simulink model "main"  (R2025b)
settings: Solver=FixedStepDiscrete  StartTime=0.0  StopTime=Inf  RelTol=1e-3  EnableMultiTasking=on
PreLoadFcn:
  | RTWConfigurationCB('preloadfcn', bdroot);
model workspace (MAT data in the model file):
  fault_count = 0
  fz_values = [0 50 100 150 200 250 300 350 400 450 500 550 600 650 700 750 800 850 900 950 1000 1050 1100 1150 1200 1250 1300 1350 1400 1450 1500 1550 1600 1650 1700 1750 1800 1850 1900 1950 2000 2050 2100]
  k_opt_lut = [0 0 0 0 0 0 0 0 0 0 0 0 ... (4386 elements, 51x2x43)]
  mu_opt_lut = [0 0 0 0 0 0 0 0 0 0 0 0 ... (4386 elements, 51x2x43)]
undefined symbols (not defined in the file or in its folder): bit, Call, Function, ocv_lut, slope_lut, soc_lut
libraries: c2837xDlib x34, c280xlib x20, canmsglib x18, c2802xlib x12, simulink x9, slpidlib x3
(part 1 of 5)
settings Model: SimulationMode=external  ExtModeTrigDuration=8  Creator=Brian  LastModifiedBy=levin
settings SolverCC: AutoInsertRateTranBlk=on
settings OptimizationCC: DefaultParameterBehavior=Inlined  DefaultUnderspecifiedDataType=single  EnhancedBackFolding=on  PassReuseOutputArgsAs=Individual arguments  MaxStackSize=1024  OptimizeBlockOrder=speed  DifferentSizesBufferReuse=on  OptimizationCustomize=off  DenormalBehavior=FlushToZero  EfficientTunableParamExpr=on
settings DebuggingCC: ParameterTunabilityLossMsg=error
settings HardwareCC: ProdBitPerChar=16.0  ProdBitPerInt=16.0  ProdBitPerPointer=32.0  ProdBitPerSizeT=32.0  ProdBitPerPtrDiffT=32.0  ProdLargestAtomicInteger=Integer  ProdLargestAtomicFloat=None  ProdWordSize=16.0  ProdLongLongMode=on  ProdHWDeviceType=Texas Instruments->C2000  HardwareBoardFeatureSet=SoCBlockset
settings ModelReferenceCC: EnableRefExpFcnMdlSchedulingChecks=on  ModelReferenceNumInstancesAllowed=Single
settings SFSimCC: MATLABDynamicMemAlloc=off
settings RTWCC: SystemTargetFile=ert.tlc  HardwareBoard=TI Delfino F28379D LaunchPad  TemplateMakefile=ert_default_tmf  Toolchain=Texas Instruments Code Composer Studio (C2000)  CodeProfilingSaveOptions=MetricsOnly  GPUComputeCapability=3.5  Description=Embedded Coder
settings CodeAppCC: ForceParamTrailComments=on  IgnoreCustomStorageClasses=off  OperatorAnnotations=on  SimulinkDataObjDesc=on  SFDataObjDesc=on  InsertBlockDesc=on
settings ERTTargetCC: ExtModeTransport=4.0  ExtModeStaticAlloc=on  ExtModeAutomaticAllocSize=off  ExtModeStaticAllocSize=10000.0  ExtModeMexFile=ext_xcp  ExtModeIntrfLevel=Level2 - Open  InlinedParameterPlacement=Hierarchical  DynamicArrayContainerType=coder::array  CodeReplacementLibrary=TI C28x  SubcomponentCodeInterfacePackaging=Nonreusable function

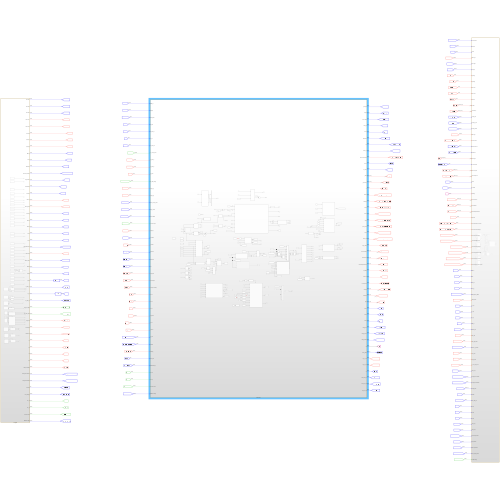
[thumbnail: Simulink's stored preview of the top-level diagram]
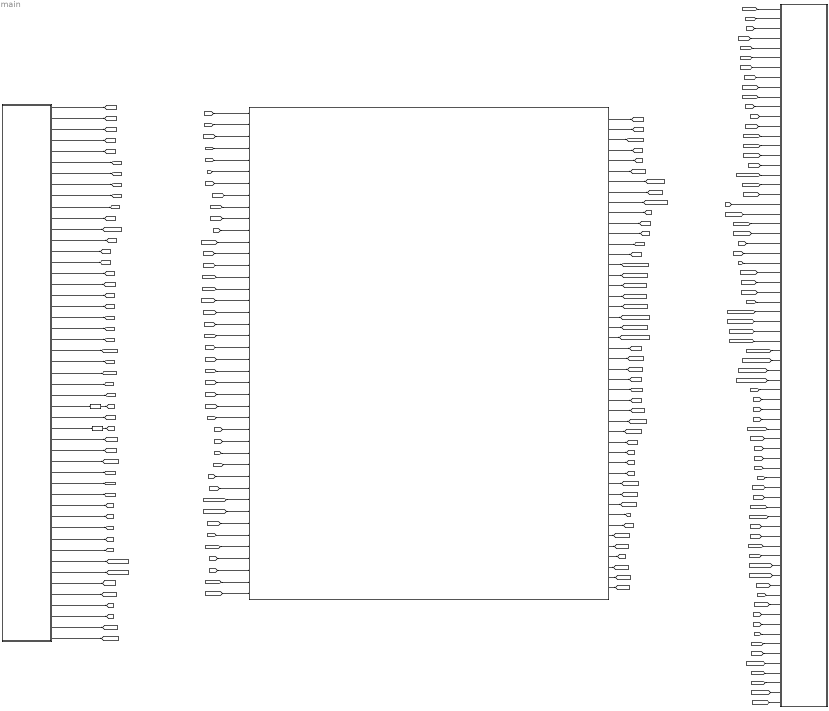
== system main ==
  Cast To Double2 : DataTypeConversion  OutDataTypeStr=uint16  SaturateOnIntegerOverflow=off  RndMeth=Floor
  Cast To Double4 : DataTypeConversion  OutDataTypeStr=uint16  SaturateOnIntegerOverflow=off  RndMeth=Floor
  In Signals : Subsystem
  MCU Code : Subsystem
  Subsystem : Subsystem
  wires:
  In Signals/5(BPT Front 2) -> [bpt_front_2]
  In Signals/20(BPT OC) -> [BPT_OC]
  In Signals/24(BSPD Fault) -> [BSPD_FAULT]
  In Signals/36(Lateral Accel) -> [Lat_Accel]
  In Signals/39(RL) -> [wss_rl]
  In Signals/29(ts_state_len) -> [ts_state_len]
  In Signals/25(Start Up Active) -> [START_UP_ACTIVE]
  In Signals/28(ts_state) -> Cast To Double2/1
  In Signals/38(FR) -> [wss_fr]
  In Signals/31(inv_state_len) -> [inv_state_len]
  In Signals/26(BMS IN) -> [BMS_IN]
  In Signals/33(inv_motor_speed) -> [inv_motor_speed]
  In Signals/40(RR) -> [wss_rr]
  In Signals/7(Apps Sig1) -> [apps_sig1]
  In Signals/3(Dash Pot 3) -> [dash_pot_3]
  In Signals/16(SDC Sig) -> [SDC_SIG]
  In Signals/17(SDC Sig Final) -> [SDC_SIG_FINAL]
  In Signals/21(CT SC) -> [CT_SC]
  In Signals/14(Screen Button) -> [screen_button]
  In Signals/37(FL) -> [wss_fl]
  In Signals/4(BPT Front 1) -> [bpt_front_1]
  In Signals/35(Accel Report) -> [accel_report]
  In Signals/27(IMD IN) -> [IMD_IN]
  In Signals/11(RTD Button) -> [RTD_Button]
  In Signals/42(Cooling Sense TB Fans) -> [Cooling_Sense_TB_Fans]
  In Signals/10(CT Sig) -> [ct_sig]
  In Signals/1(Dash Pot 1) -> [dash_pot_1]
  In Signals/2(Dash Pot 2) -> [dash_pot_2]
  In Signals/8(Apps Sig2) -> [apps_sig2]
  In Signals/34(Long Accel) -> [Long_Accel]
  MCU Code/31(Out-Speed) -> [MoTec_Out_Speec]
  MCU Code/4(ready_led) -> [RTD_LED]
  MCU Code/17(enable) -> [VCU_INV_Inverter_Enable]
  [RTD_Button] -> MCU Code/3(RTD_Button)
  [ts_state_len] -> MCU Code/5(ts_state_len)
  [LV_Vehicle_State] -> Subsystem/22(LV Vehicle State)
  MCU Code/14(Out18) -> [Brake_Light]
  [VCU_INV_Torque_Command] -> Subsystem/38(VCU INV Torque Command)
  In Signals/19(BPT SC) -> [BPT_SC]
  [cooling_tb_fans] -> Subsystem/15(Cooling_tb_fans)
  MCU Code/35(Knob3) -> [Knob3]
  [Knob3] -> Subsystem/65(Knob3)
  MCU Code/28(driver cmd) -> [driver_cmd]
  [Accel_Estimate] -> Subsystem/29(Accel Estimate)
  [Inverter_Enable] -> Subsystem/1(Inverter Enable)
  [dash_pot_3] -> MCU Code/24(In26)
  MCU Code/25(Accel Estimate) -> [Accel_Estimate]
  [Lights] -> Subsystem/21(Dash Lights)
  [CT_OC] -> Subsystem/46(CT_OC)
  [Regen_State] -> Subsystem/55(Regen_State)
  [cooling_loop] -> Subsystem/14(Cooling_loop)
  MCU Code/18(counter) -> [VCU_INV_Rolling_Counter]
  [apps_sig2] -> Subsystem/8(Apps Sig2)
  MCU Code/33(Knob1) -> [Knob1]
  [SDC_SIG] -> Subsystem/51(SDC_SIG)
  [Screen] -> Subsystem/25(Screen)
  MCU Code/27(Slip Ratio) -> [Slip_Ratio]
  [RTD_LED] -> Subsystem/2(RTD LED)
  [BSPD_DUAL_CHECK] -> Subsystem/44(BSPD_DUAL_CHECK)
  [apps_sig1] -> Subsystem/7(Apps Sig1)
  [SDC_SIG_FINAL] -> Subsystem/52(SDC_SIG_FINAL)
  MCU Code/20(speed_mode) -> [VCU_INV_Speed_Mode_Enable]
  [LV_Echo_TS_State] -> Subsystem/19(TS State Timeout)
  [Regen_switch] -> MCU Code/16(Regen_switch)
  [dis] -> Subsystem/27(discharge)
  [Long_Accel] -> MCU Code/25(Long Accel)
  MCU Code/26(Forward Speed Estimate) -> [Fwd_Speed_Est]
  [START_UP_ACTIVE] -> Subsystem/53(START_UP_ACTIVE)
  MCU Code/5(buzzer) -> [Buzzer]
  [Long_Accel] -> MCU Code/31(long accel)
  [r_momentary] -> Subsystem/13(R Momentary)
  [DC_Bus_Voltage] -> MCU Code/12(DC_Bus_Voltage)
  MCU Code/23(Regen_State) -> [Regen_State]
  In Signals/22(CT OC) -> [CT_OC]
  [Error_Covariance] -> Subsystem/28(Error Covariance)
  [dash_pot_1] -> MCU Code/22(Dash Pot 1)
  [cooling_radiator] -> Subsystem/16(Cooling_radiator)
  [Buzzer] -> Subsystem/3(Buzzer)
  [accel_report] -> MCU Code/26(Accel Report)
  MCU Code/13(r_momentary) -> [r_momentary]
  [VCU_INV_Speed_Mode_Enable] -> Subsystem/37(VCU INV Speed Mode Enable)
  MCU Code/11(TC_switch) -> [TC_switch]
  MCU Code/32(lights) -> [Lights]
  [inv_motor_speed] -> MCU Code/8(inv_ motor_speed)
  [inv_motor_speed] -> MCU Code/18(inv motor speed)
  [screen_button] -> MCU Code/17(Screen Button)
  MCU Code/38(cooling_radiator) -> [cooling_radiator]
  MCU Code/36(cooling_loop) -> [cooling_loop]
  [VCU_INV_Rolling_Counter] -> Subsystem/35(VCU INV Rolling Counter)
  In Signals/6(BPT Rear) -> [bpt_rear]
  [BMS_IN] -> Subsystem/40(BMS In)
  [BPT_OC] -> Subsystem/41(BPT)
  [apps_sig1] -> MCU Code/19(apps sig1)
  [VCU_INV_Direction_Command] -> Subsystem/32(VCU INV Direction Command)
  [cooling_faults] -> Subsystem/60(cooling_faults)
  [dash_pot_3] -> Subsystem/57(dash_pot_3)
  Cast To Double4/1 -> [inv_en]
  [Brake_Light] -> Subsystem/4(Brake Light)
  [bpt_front_1] -> MCU Code/9(bpt_front_1)
  [Red_Light] -> Subsystem/6(Red Light)
  MCU Code/19(speed) -> [VCU_INV_Speed_Command]
  [inv_state_len] -> MCU Code/7(inv_state_len)
  [dash_pot_2] -> Subsystem/67(dash_pot_2)
  [Slip_Ratio] -> Subsystem/31(Slip Ratio)
  [Cooling_Sense_Radiator] -> Subsystem/59(Cooling Sense Radiator)
  MCU Code/8(inverter_en) -> [Inverter_Enable]
  MCU Code/6(RTD Button) -> [LV_RTD_Button]
  [MoTec_In_Speed] -> Subsystem/23(MoTec In Speed)
  MCU Code/22(torque_limit) -> [VCU_INV_Torque_Limit_Command]
  In Signals/30(inv_en) -> Cast To Double4/1
  MCU Code/24(Error Covariance) -> [Error_Covariance]
  [bse_sig] -> Subsystem/43(bse_sig)
  [driver_cmd] -> Subsystem/54(driver_cmd)
  Cast To Double2/1 -> [ts_state]
  MCU Code/29(TC Torque Cmd) -> [LV_TC_Torque_Cmd]
  [Cooling_Sense_TB_Fans] -> Subsystem/58(Cooling Sense TB Fans)
  [wss_rr] -> MCU Code/32(wss rr)
  MCU Code/30(In-Speed) -> [MoTec_In_Speed]
  MCU Code/16(discharge) -> [VCU_INV_Inverter_Discharge]
  MCU Code/12(r_faults) -> [r_faults]
  [VCU_INV_Inverter_Enable] -> Subsystem/34(VCU INV Inverter Enable)
  In Signals/9(BSE Sig) -> [bse_sig]
  [dash_pot_1] -> Subsystem/66(dash_pot_1)
  [Lat_Accel] -> MCU Code/21(Lat Accel)
  MCU Code/1(green light) -> [Green_Light]
  In Signals/41(Velocity Timestamp) -> [vel_time]
  In Signals/13(Regen Switch) -> [Regen_switch]
  [IMD_IN] -> Subsystem/49(IMD_IN)
  [IMD_IN] -> MCU Code/2(IMD_IN)
  MCU Code/40(cooling_faults) -> [cooling_faults]
  [LV_RTD_Button] -> Subsystem/20(RTD Button)
  [MoTec_Out_Speec] -> Subsystem/24(MoTec Out Speed)
  [ct_sig] -> Subsystem/48(ct_sig)
  [Lat_Accel] -> MCU Code/33(lat accel)
  In Signals/23(BSPD Dual Check) -> [BSPD_DUAL_CHECK]
  MCU Code/21(torque) -> [VCU_INV_Torque_Command]
  [BSPD_FAULT] -> Subsystem/45(BSPD_FAULT)
  [Cooling_Sense_Radiator] -> MCU Code/35(radiator)
  [LV_Echo_Inverter_Enable] -> Subsystem/18(Inverter enable)
  [LV_TC_Torque_Cmd] -> Subsystem/56(LV_TC_Torque_Cmd)
  [vel_time] -> MCU Code/27(Velocity Timestamp)
  [BPT_SC] -> Subsystem/42(BPT_SC)
  MCU Code/39(dis) -> [dis]
  In Signals/43(Cooling Sense Raditor) -> [Cooling_Sense_Radiator]
  [Knob1] -> Subsystem/63(Knob1)
  [TC_button] -> MCU Code/20(TC Button)
  [RESET_SIG] -> Subsystem/50(RESET_SIG)
  [bpt_rear] -> Subsystem/11(BPT Rear)
  [Knob2] -> Subsystem/64(Knob2)
  [bpt_front_1] -> Subsystem/9(BPT Front 1)
  [ts_state] -> MCU Code/4(ts_state)
  MCU Code/37(cooling_tb_fans) -> [cooling_tb_fans]
  [VCU_INV_Speed_Command] -> Subsystem/36(VCU INV Speed Command)
  In Signals/15(TC Button) -> [TC_button]
  [Driver_torque_switch] -> MCU Code/15(Driver_Torque_switch)
  [bpt_front_2] -> MCU Code/10(bpt_front_2)
  [Fwd_Speed_Est] -> Subsystem/30(Forward Speed Estimate)
  [dash_pot_2] -> MCU Code/23(Dash Pot 2)
  [Brake_Light] -> Subsystem/17(Brake light)
  [apps_sig2] -> MCU Code/14(apps_sig2)
  [Green_Light] -> Subsystem/5(Green Light)
  MCU Code/3(Vehicle State) -> [LV_Vehicle_State]
  [wss_fl] -> MCU Code/28(wss fl)
  MCU Code/15(direction) -> [VCU_INV_Direction_Command]
  MCU Code/7(out) -> [LV_Echo_TS_State]
  [TC_switch] -> Subsystem/26(TC Switch)
  MCU Code/9(Echo Inverter Enable) -> [LV_Echo_Inverter_Enable]
  [apps_sig1] -> MCU Code/13(apps_sig1)
  MCU Code/34(Knob2) -> [Knob2]
  [VCU_INV_Inverter_Discharge] -> Subsystem/33(VCU INV Inverter Discharge)
  [wss_rl] -> MCU Code/30(wss rl)
  In Signals/32(DC_Bus_Voltage) -> [DC_Bus_Voltage]
  [VCU_INV_Torque_Limit_Command] -> Subsystem/39(VCU INV Torque Limit Command)
  In Signals/18(Reset Sig) -> [RESET_SIG]
  [wss_fr] -> MCU Code/29(wss fr)
  [BMS_IN] -> MCU Code/1(BMS_IN)
  [bpt_rear] -> MCU Code/11(bpt_rear)
  [inv_en] -> MCU Code/6(inv_en)
  In Signals/12(Driver Torque Switch) -> [Driver_torque_switch]
  [CT_SC] -> Subsystem/47(CT_SC)
  MCU Code/10(Screen) -> [Screen]
  MCU Code/2(red light) -> [Red_Light]
  [r_faults] -> Subsystem/12(R Faults)
  [Cooling_Sense_TB_Fans] -> MCU Code/34(tb_fans)
  MCU Code/41(bpt_f_1_bar) -> [bpt_front_bar_1]
  MCU Code/42(bpt_f_2_bar) -> [bpt_front_bar_2]
  [bpt_front_2] -> Subsystem/10(BPT Front 2)
  [SDC_SIG_FINAL] -> MCU Code/36(SDC Sig)
  In Signals/44(RX DATA) -> [RXData]
  [RXData] -> MCU Code/37(Servo_Pos)
  MCU Code/43(TX) -> [TXData]
  [TXData] -> Subsystem/61(TXData)
  MCU Code/44(brake_bias_pos) -> [brake_bias_pos]
  [brake_bias_pos] -> Subsystem/62(brake_bias_pos)
  [Driver_torque_switch] -> Subsystem/68(Driver Torque Switch)
  [Regen_switch] -> Subsystem/69(Regen Switch)
  In Signals/45(bsm_discharge) -> [BSM_Discharge]
  [BSM_Discharge] -> MCU Code/38(BSM Discharge)
  MCU Code/45(driver_input_ctrl) -> [driver_input_ctrl]
  MCU Code/46(mcu_input_ctrl) -> [mcu_input_ctrl]
  [mcu_input_ctrl] -> Subsystem/70(MCU Input Control)
  [Driver_torque_switch] -> Subsystem/71(Driver_Torque_Switch)
  In Signals/46(INV_Id) -> [INV_Id]
  In Signals/47(INV_Iq) -> [INV_Iq]
  [INV_Iq] -> MCU Code/40(INV Iq)
  [INV_Id] -> MCU Code/39(INV Id)
  In Signals/48(DC Bus Current) -> [DC_Bus_Current]
  [DC_Bus_Current] -> MCU Code/41(DC Bus Current)
  [DC_Bus_Voltage] -> Subsystem/72(DC Bus Voltage)
  In Signals/49(BMS Min Voltage) -> [BMS_Min_Voltage]
  [BMS_Min_Voltage] -> MCU Code/42(BMS Min Voltage)
